simulink model "sim_discrete_7dof"  (R2022b)
settings: Solver=VariableStepAuto  StartTime=0.0  StopTime=T_sim  FixedStep=param_global.Ta  RelTol=1e-3
InitFcn:
  | parameters_7dof;
undefined symbols (not defined in the file): fx, fy, fz, init_bus_param, MPC9, n, param_global, param_robot, param_savgol, param_vis, tau_x, tau_y, tau_z, v4_kin_int_refsys
settings Model: Creator=emu  LastModifiedBy=emu
settings OptimizationCC: ReuseModelBlockBuffer=on
settings DebuggingCC: ReadBeforeWriteMsg=DisableAll  WriteAfterWriteMsg=DisableAll  WriteAfterReadMsg=DisableAll  MultiTaskDSMMsg=none
settings ModelReferenceCC: UpdateModelReferenceTargets=IfOutOfDate
settings SFSimCC: SFSimEcho=off
settings ExplorerConfigSet: InternalSimMechanicsExplorerSettings="<ExplorerConfiguration><canonicalview>default</canonicalview><AnimationSetting><BasePlaybackSpeed>1.0</BasePlaybackSpeed><PlaybackSpeedFactor>1.0</PlaybackSpeedFactor></AnimationSetting><TilePanel><TileInfo><Tiles Columns=\"1\" Count=\"1\" Rows=\"1\"><Column Weight=\"1\"/><Row Weight=\"1\"/><Tile Height=\"1\" Width=\"1\" X=\"0\" Y=\"0\"/></Tiles></TileInfo><SceneInfo><SceneViewer><BGColor><R>0.60000002384185791</R><G>0.60000002384185791</G><B>0.60000002384185791</B></BGColor><Camera><DoPerspective>off</DoPerspective><Position><X>0.252311079271715533</X><Y>1.1744281053543093</Y><Z>0.804106796949367042</Z></Position><Center><X>0.252311079271715533</X><Y>0.174428105354309249</Y><Z>0.804106796949367042</Z></Center><Up><X>0</X><Y>0</Y><Z>1</Z></Up><ViewLimDist>1</ViewLimDist><YLim>0.464787140947337862</YLim><XLim>0.887662117098616976</XLim></Camera></SceneViewer></SceneInfo></TilePanel><MechEditorPanel><Cameras/><GfxPanelCameraMap/><VideoCreator><PlaybackSpeedRatio>1.0</PlaybackSpeedRatio><FrameRate>30</FrameRate><VideoFormat>Motion JPEG AVI</VideoFormat><FrameSize>auto</FrameSize></VideoCreator></MechEditorPanel></ExplorerConfiguration>"

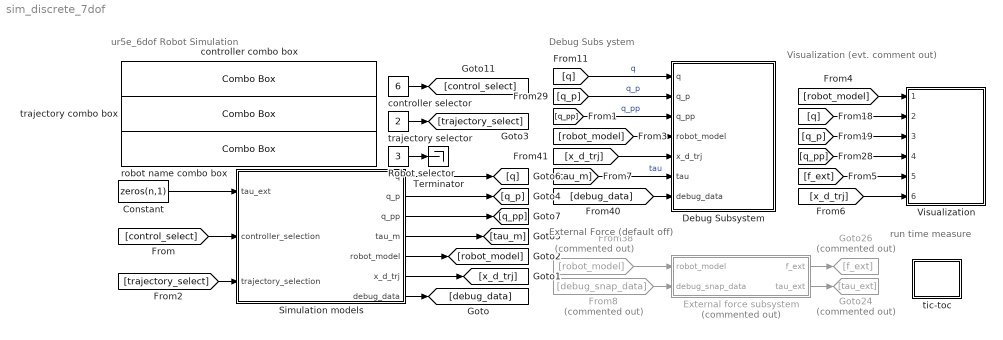
== system sim_discrete_7dof ==
  note: run time measure
  note: ur5e_6dof Robot Simulation
  note: Visualization (evt. comment out)
  note: Debug Subs ystem
  note: External Force (default off)
  Constant : Constant  Value=zeros(n,1)
  Debug Subsystem : Subsystem
  External force subsystem : Subsystem  Commented=on
  From38 : From  Commented=on  GotoTag=robot_model
  From8 : From  Commented=on  GotoTag=debug_snap_data
  Goto24 : Goto  Commented=on  GotoTag=tau_ext
  Goto26 : Goto  Commented=on  GotoTag=f_ext
  Robot selector : Constant  Value=3
  Simulation models : Subsystem
  Terminator : Terminator
  Visualization : Subsystem  ReferencedSubsystem=Visualization_shared_subsystem
  controller combo box : ComboBox  SelectedLabel=MPC9 (v4_kin_int_refsys)
      settings: Values={{'Cartesian CT Control', 'MPC01', 'MPC6 (v3_quat)', 'MPC7 (v3_rpy)', 'MPC8 (v4_kin_int)', 'MPC9 (v4_kin_int_refsys)', 'MPC10 (v5_kin_dev)'}, [1 2 3 4 5 6 7]}
  controller selector : Constant  Value=6  OutDataTypeStr=uint32  SampleTime=-1
  robot name combo box : ComboBox  SelectedLabel=ur5e_6dof
      settings: Values={{'fr3_7dof', 'fr3_6dof', 'ur5e_6dof'}, [1 2 3]}
  tic-toc : Subsystem
  trajectory combo box : ComboBox  SelectedLabel=2: Allsingularity, Polynomial, Workspace
      settings: Values={{'1: Wrist Singularity 1, Polynomial, Workspace', '2: Allsingularity, Polynomial, Workspace', '3: Ellbow Singularity 1, Polynomial, Workspace', '4: ELLBOW Singularity 2, Polynomial, Workspace', '5: ELLBOW Singularity 2, Polynomial, joint space', '6: Shoulder Singularity, Polynomial, Workspace', '7: Shoulder Sing 2, Polynomial, Workspace'}, [1 2 3 4 5 6 7]}
  trajectory selector : Constant  Value=2  OutDataTypeStr=uint32  SampleTime=-1
  wires:
  controller selector/1 -> [control_select]
  [tau_m] -> Debug Subsystem/6(tau)  "tau"
  [debug_data] -> Debug Subsystem/7(debug_data)
  External force subsystem/1(f_ext) -> Goto26/1
  [q_p] -> Debug Subsystem/2(q_p)  "q_p"
  [robot_model] -> Debug Subsystem/4(robot_model)
  [robot_model] -> Visualization/1
  From8/1 -> External force subsystem/2(debug_snap_data)
  [q_pp] -> Visualization/4
  [f_ext] -> Visualization/5
  [x_d_trj] -> Debug Subsystem/5(x_d_trj)
  From38/1 -> External force subsystem/1(robot_model)
  [q_p] -> Visualization/3
  External force subsystem/2(tau_ext) -> Goto24/1
  [q] -> Visualization/2
  [q] -> Debug Subsystem/1(q)  "q"
  [q_pp] -> Debug Subsystem/3(q_pp)  "q_pp"
  Simulation models/7(debug_data) -> [debug_data]
  Simulation models/6(x_d_trj) -> [x_d_trj]
  Simulation models/5(robot_model) -> [robot_model]
  Simulation models/4(tau_m) -> [tau_m]
  Simulation models/3(q_pp) -> [q_pp]
  Simulation models/2(q_p) -> [q_p]
  Simulation models/1(q) -> [q]
  [control_select] -> Simulation models/2(controller_selection)
  Constant/1 -> Simulation models/1(tau_ext)
  trajectory selector/1 -> [trajectory_select]
  [trajectory_select] -> Simulation models/3(trajectory_selection)
  Robot selector/1 -> Terminator/1
  [x_d_trj] -> Visualization/6

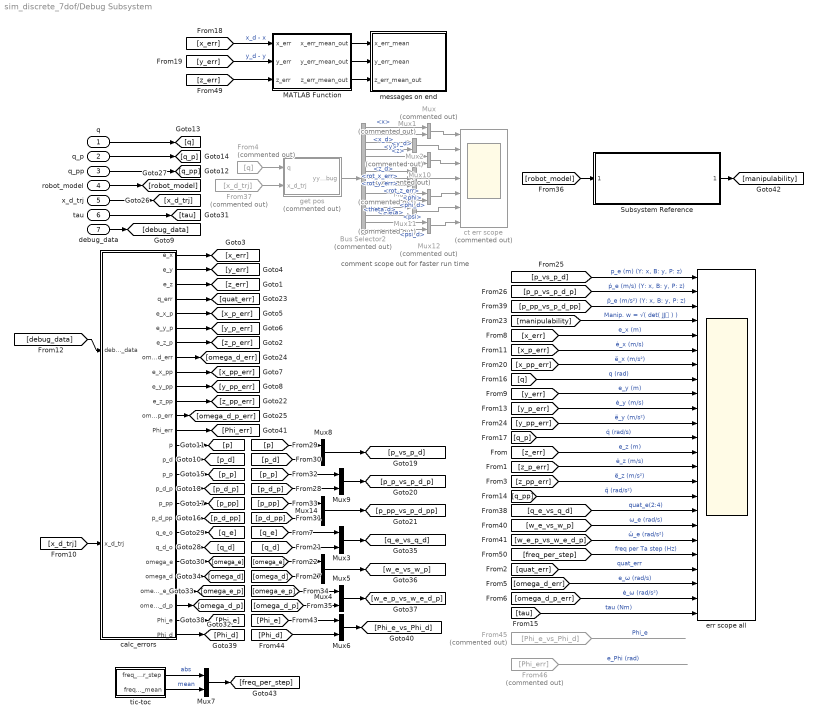
== system sim_discrete_7dof/Debug Subsystem ==
  note: comment scope out for faster run time
  q : Inport
  q_p : Inport  Port=2
  q_pp : Inport  Port=3
  robot_model : Inport  Port=4
  x_d_trj : Inport  Port=5
  tau : Inport  Port=6
  debug_data : Inport  Port=7  OutDataTypeStr=Bus: debug_data_bus
  Bus Selector2 : BusSelector  Commented=on  OutputSignals=x,x_d,y,y_d,z,z_d,rot_x_err,rot_y_err,rot_z_err,phi,phi_d,theta,theta_d,psi,psi_d
  From37 : From  Commented=on  GotoTag=x_d_trj
  From4 : From  Commented=on  GotoTag=q
  From45 : From  Commented=on  GotoTag=Phi_e_vs_Phi_d
  From46 : From  Commented=on  GotoTag=Phi_err
  MATLAB Function : MATLAB Function  TreatAsAtomicUnit=on
  Mux{,1..2,10..12} (6 alike) : Mux  Commented=on  Inputs=2
  Mux13 : Mux  Commented=on  Inputs=3
  Mux{3..9,14} (8 alike) : Mux  Inputs=2
  Subsystem Reference : Subsystem  ReferencedSubsystem=manipulability_and_collinearity
  calc_errors : MATLAB Function  TreatAsAtomicUnit=on
  ct err scope : Scope  Commented=on  NumInputPorts=7
  err scope all : Scope  NumInputPorts=24
  get pos : MATLAB Function  Commented=on  TreatAsAtomicUnit=on  SystemSampleTime=param_global.Ta
  messages on end : Subsystem
  tic-toc : Subsystem
  wires:
  q/1 -> [q]
  q_p/1 -> [q_p]
  q_pp/1 -> [q_pp]
  From4/1 -> get pos/1(q)
  x_d_trj/1 -> [x_d_trj]
  robot_model/1 -> [robot_model]
  debug_data/1 -> [debug_data]
  tau/1 -> [tau]
  From37/1 -> get pos/2(x_d_trj)
  get pos/1(yy_debug) -> Bus Selector2/1
  Mux/1 -> ct err scope/1
  Mux1/1 -> ct err scope/2
  Mux2/1 -> ct err scope/3
  Mux10/1 -> ct err scope/5
  Mux11/1 -> ct err scope/6
  Mux12/1 -> ct err scope/7
  Mux13/1 -> ct err scope/4
  Bus Selector2/1 -> Mux/1  "<x>"
  Bus Selector2/2 -> Mux/2  "<x_d>"
  Bus Selector2/3 -> Mux1/1  "<y>"
  Bus Selector2/4 -> Mux1/2  "<y_d>"
  Bus Selector2/5 -> Mux2/1  "<z>"
  Bus Selector2/6 -> Mux2/2  "<z_d>"
  Bus Selector2/7 -> Mux13/1  "<rot_x_err>"
  Bus Selector2/8 -> Mux13/2  "<rot_y_err>"
  Bus Selector2/9 -> Mux13/3  "<rot_z_err>"
  Bus Selector2/10 -> Mux10/1  "<phi>"
  Bus Selector2/11 -> Mux10/2  "<phi_d>"
  Bus Selector2/12 -> Mux11/1  "<theta>"
  Bus Selector2/13 -> Mux11/2  "<theta_d>"
  Bus Selector2/14 -> Mux12/1  "<psi>"
  Bus Selector2/15 -> Mux12/2  "<psi_d>"
  [x_err] -> MATLAB Function/1(x_err)  "x_d - x"
  [y_err] -> MATLAB Function/2(y_err)  "y_d - y"
  MATLAB Function/2(y_err_mean_out) -> messages on end/2(y_err_mean)
  MATLAB Function/1(x_err_mean_out) -> messages on end/1(x_err_mean)
  [debug_data] -> calc_errors/1(debug_data)
  [x_d_trj] -> calc_errors/2(x_d_trj)
  calc_errors/1(e_x) -> [x_err]
  calc_errors/2(e_y) -> [y_err]
  calc_errors/5(e_x_p) -> [x_p_err]
  calc_errors/6(e_y_p) -> [y_p_err]
  calc_errors/9(e_x_pp) -> [x_pp_err]
  calc_errors/10(e_y_pp) -> [y_pp_err]
  [manipulability] -> err scope all/4  "Manip. w = √( det( JJ⸆ ) )"
  [tau] -> err scope all/24  "tau (Nm)"
  [x_err] -> err scope all/5  "e_x (m)"
  [y_err] -> err scope all/9  "e_y (m)"
  [x_p_err] -> err scope all/6  "ė_x (m/s)"
  [y_p_err] -> err scope all/10  "ė_y (m/s)"
  [x_pp_err] -> err scope all/7  "ё_x (m/s²)"
  [y_pp_err] -> err scope all/11  "ё_y (m/s²)"
  [q] -> err scope all/8  "q (rad)"
  [q_p] -> err scope all/12  "q̇ (rad/s)"
  [q_pp] -> err scope all/16  "q̈ (rad/s²)"
  [p_d_p] -> Mux9/2
  [p_p] -> Mux9/1
  [p_d] -> Mux8/2
  [p] -> Mux8/1
  [p_pp] -> Mux14/1
  [p_d_pp] -> Mux14/2
  [p_p_vs_p_d_p] -> err scope all/2  "ṗ_e (m/s) (Y: x, B: y, P: z)"
  [p_vs_p_d] -> err scope all/1  "p_e (m) (Y: x, B: y, P: z)"
  [p_pp_vs_p_d_pp] -> err scope all/3  "p̈_e (m/s²) (Y: x, B: y, P: z)"
  Mux8/1 -> [p_vs_p_d]
  Mux9/1 -> [p_p_vs_p_d_p]
  Mux14/1 -> [p_pp_vs_p_d_pp]
  calc_errors/14(p) -> [p]
  calc_errors/15(p_d) -> [p_d]
  calc_errors/16(p_p) -> [p_p]
  calc_errors/17(p_d_p) -> [p_d_p]
  calc_errors/18(p_pp) -> [p_pp]
  calc_errors/19(p_d_pp) -> [p_d_pp]
  calc_errors/3(e_z) -> [z_err]
  calc_errors/7(e_z_p) -> [z_p_err]
  calc_errors/11(e_z_pp) -> [z_pp_err]
  [z_err] -> err scope all/13  "e_z (m)"
  [z_p_err] -> err scope all/14  "ė_z (m/s)"
  [z_pp_err] -> err scope all/15  "ё_z (m/s²)"
  calc_errors/4(q_err) -> [quat_err]
  calc_errors/12(omega_d_p_err) -> [omega_d_p_err]
  calc_errors/8(omega_d_err) -> [omega_d_err]
  [quat_err] -> err scope all/21  "quat_err"
  [omega_d_err] -> err scope all/22  "e_ω (rad/s)"
  [omega_d_p_err] -> err scope all/23  "ė_ω (rad/s²)"
  calc_errors/20(q_e_o) -> [q_e]
  calc_errors/21(q_d_o) -> [q_d]
  calc_errors/22(omega_e) -> [omega_e]
  calc_errors/23(omega_d) -> [omega_d]
  calc_errors/24(omega_e_p) -> [omega_e_p]
  calc_errors/25(omega_d_p) -> [omega_d_p]
  [q_e] -> Mux3/1
  [q_d] -> Mux3/2
  [omega_e] -> Mux4/1
  [omega_d] -> Mux4/2
  [omega_e_p] -> Mux5/1
  [omega_d_p] -> Mux5/2
  Mux3/1 -> [q_e_vs_q_d]
  Mux4/1 -> [w_e_vs_w_p]
  Mux5/1 -> [w_e_p_vs_w_e_d_p]
  [q_e_vs_q_d] -> err scope all/17  "quat_e(2:4)"
  [w_e_vs_w_p] -> err scope all/18  "ω_e (rad/s)"
  [w_e_p_vs_w_e_d_p] -> err scope all/19  "ὠ_e (rad/s²)"
  calc_errors/26(Phi_e) -> [Phi_e]
  calc_errors/27(Phi_d) -> [Phi_d]
  [Phi_d] -> Mux6/2
  [Phi_e] -> Mux6/1
  Mux6/1 -> [Phi_e_vs_Phi_d]
  From45/1 -> ?  "Phi_e"
  calc_errors/13(Phi_err) -> [Phi_err]
  From46/1 -> ?  "e_Phi (rad)"
  [z_err] -> MATLAB Function/3(z_err)
  MATLAB Function/3(z_err_mean_out) -> messages on end/3(z_err_mean_out)
  [freq_per_step] -> err scope all/20  "freq per Ta step (Hz)"
  Subsystem Reference/1 -> [manipulability]
  [robot_model] -> Subsystem Reference/1
  Mux7/1 -> [freq_per_step]
  tic-toc/1(freq_per_step) -> Mux7/1  "abs"
  tic-toc/2(freq_per_step_mean) -> Mux7/2  "mean"

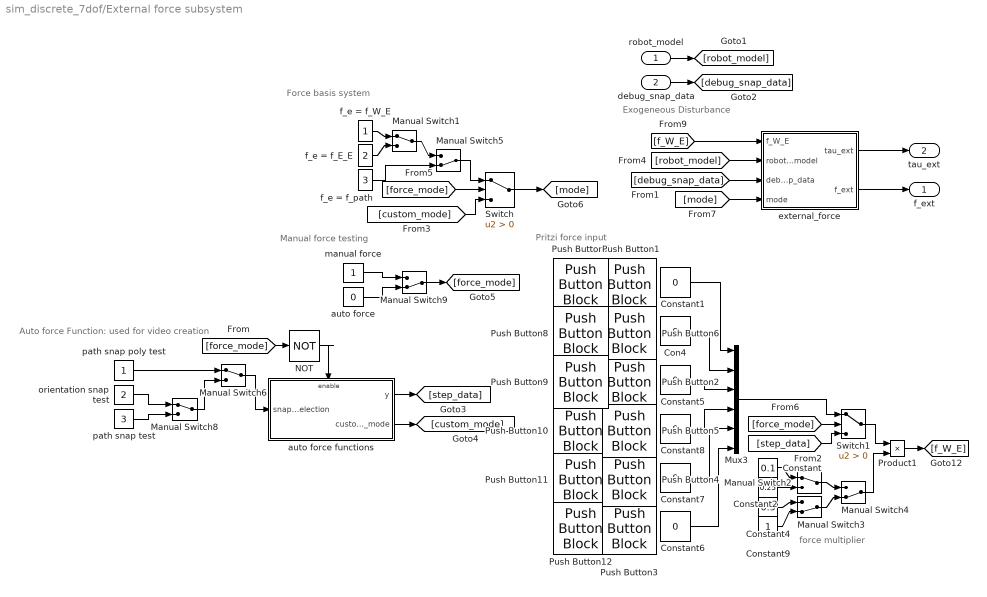
== system sim_discrete_7dof/External force subsystem ==
  note: Force basis system
  note: Manual force testing
  note: Auto force Function: used for video creation
  note: force multiplier
  note: Exogeneous Disturbance
  note: Pritzi force input
  robot_model : Inport
  debug_snap_data : Inport  Port=2  OutDataTypeStr=Bus: debug_snap_data_bus
  Con4 : Constant  Value=0  SampleTime=-1
  Constant : Constant  Value=0.1  SampleTime=-1
  Constant{1,5..8} (5 alike) : Constant  Value=0  SampleTime=-1
  Constant2 : Constant  Value=0.25  SampleTime=-1
  Constant4 : Constant  Value=0.5  SampleTime=-1
  Constant9 : Constant  SampleTime=-1
  Manual Switch{1..2,6,8} (4 alike) : ManualSwitch
  Manual Switch{3..5,9} (4 alike) : ManualSwitch  CurrentSetting=0
  Mux3 : Mux  Inputs=6
  NOT : Logic  Operator=NOT  IconShape=distinctive  AllPortsSameDT=off  OutDataTypeStr=boolean
  Product1 : Product
  Push Button1 : PushButtonBlock  ButtonText=fx  OnValue=20  OffValue=0.000000
  Push Button10 : PushButtonBlock  ButtonText=-tau_x  OnValue=-1  OffValue=0.000000
  Push Button11 : PushButtonBlock  ButtonText=-tau_y  OnValue=-1  OffValue=0.000000
  Push Button12 : PushButtonBlock  ButtonText=-tau_z  OnValue=-1  OffValue=0.000000
  Push Button2 : PushButtonBlock  ButtonText=fz  OnValue=20  OffValue=0.000000
  Push Button3 : PushButtonBlock  ButtonText=tau_z  OffValue=0.000000
  Push Button4 : PushButtonBlock  ButtonText=tau_y  OffValue=0.000000
  Push Button5 : PushButtonBlock  ButtonText=tau_x  OffValue=0.000000
  Push Button6 : PushButtonBlock  ButtonText=fy  OnValue=20  OffValue=0.000000
  Push Button7 : PushButtonBlock  ButtonText=-fx  OnValue=-20  OffValue=0.000000
  Push Button8 : PushButtonBlock  ButtonText=-fy  OnValue=-20  OffValue=0.000000
  Push Button9 : PushButtonBlock  ButtonText=-fz  OnValue=-20  OffValue=0.000000
  Switch : Switch  Criteria=u2 > Threshold  SaturateOnIntegerOverflow=off  InputSameDT=off
  Switch1 : Switch  Criteria=u2 > Threshold  SaturateOnIntegerOverflow=off  InputSameDT=off
  auto force : Constant  Value=0
  auto force functions : Subsystem
  external_force : MATLAB Function  TreatAsAtomicUnit=on
  f_e = f_E_E : Constant  Value=2  SampleTime=-1
  f_e = f_W_E : Constant  SampleTime=-1
  f_e = f_path : Constant  Value=3  SampleTime=-1
  manual force : Constant
  orientation snap test : Constant  Value=2
  path snap poly test : Constant
  path snap test : Constant  Value=3
  f_ext : Outport
  tau_ext : Outport  Port=2
  wires:
  Product1/1 -> [f_W_E]
  Constant4/1 -> Manual Switch3/1
  Constant6/1 -> Mux3/6
  Constant5/1 -> Mux3/3
  Constant/1 -> Manual Switch2/1
  Constant8/1 -> Mux3/4
  [f_W_E] -> external_force/1(f_W_E)
  external_force/2(f_ext) -> f_ext/1
  Constant9/1 -> Manual Switch3/2
  Manual Switch2/1 -> Manual Switch4/1
  Con4/1 -> Mux3/2
  [robot_model] -> external_force/2(robot_model)
  Manual Switch4/1 -> Product1/2
  Constant1/1 -> Mux3/1
  f_e = f_W_E/1 -> Manual Switch1/1
  Constant7/1 -> Mux3/5
  Constant2/1 -> Manual Switch2/2
  f_e = f_E_E/1 -> Manual Switch1/2
  Manual Switch3/1 -> Manual Switch4/2
  external_force/1(tau_ext) -> tau_ext/1
  Manual Switch1/1 -> Manual Switch5/1
  f_e = f_path/1 -> Manual Switch5/2
  robot_model/1 -> [robot_model]
  debug_snap_data/1 -> [debug_snap_data]
  [debug_snap_data] -> external_force/3(debug_snap_data)
  Switch1/1 -> Product1/1
  Manual Switch5/1 -> Switch/1
  [custom_mode] -> Switch/3
  auto force functions/1(y) -> [step_data]
  auto force functions/2(custom_mode) -> [custom_mode]
  Manual Switch6/1 -> auto force functions/1(snap selection)
  path snap test/1 -> Manual Switch8/2
  orientation snap test/1 -> Manual Switch8/1
  manual force/1 -> Manual Switch9/1
  auto force/1 -> Manual Switch9/2
  Manual Switch9/1 -> [force_mode]
  [force_mode] -> Switch/2
  [force_mode] -> Switch1/2
  [step_data] -> Switch1/3
  Mux3/1 -> Switch1/1
  Switch/1 -> [mode]
  [mode] -> external_force/4(mode)
  Manual Switch8/1 -> Manual Switch6/2
  path snap poly test/1 -> Manual Switch6/1
  [force_mode] -> NOT/1
  NOT/1 -> auto force functions/Enable

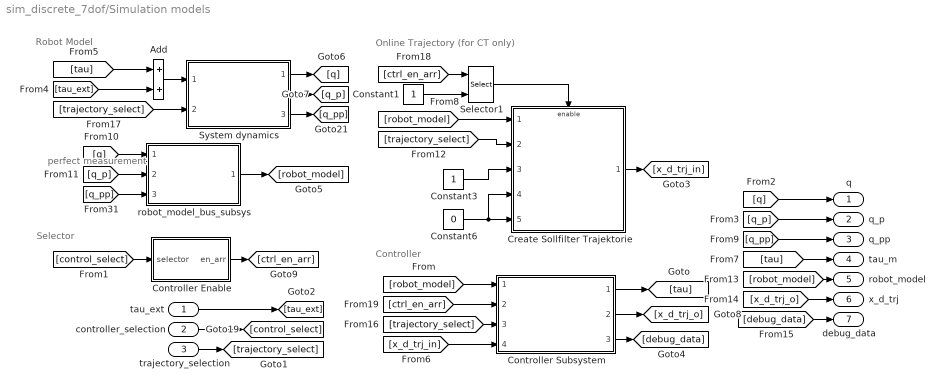
== system sim_discrete_7dof/Simulation models ==
  note: Selector
  note: Controller
  note: Online Trajectory (for CT only)
  note: Robot Model
  note: perfect measurement
  tau_ext : Inport
  controller_selection : Inport  Port=2
  trajectory_selection : Inport  Port=3
  Add : Sum
  Constant1 : Constant
  Constant3 : Constant
  Constant6 : Constant  Value=0
  Controller Enable : MATLAB Function  TreatAsAtomicUnit=on
  Controller Subsystem : Subsystem  ReferencedSubsystem=controller_ref_subsys
  Create Sollfilter Trajektorie : Subsystem  ReferencedSubsystem=trajectory_generation_ref_subsys_7dof
  Selector1 : Selector  IndexOptions=Index vector (port)  Indices=[1 3]  OutputSizes=1
  System dynamics : Subsystem  ReferencedSubsystem=robot_model_7dof_ref_subsys
  robot_model_bus_subsys : Subsystem  ReferencedSubsystem=robot_model_bus_7dof_ref_subsys
  q : Outport
  q_p : Outport  Port=2
  q_pp : Outport  Port=3
  tau_m : Outport  Port=4
  robot_model : Outport  Port=5  OutDataTypeStr=Bus: robot_model
  x_d_trj : Outport  Port=6  OutDataTypeStr=Bus: x_d
  debug_data : Outport  Port=7  OutDataTypeStr=Bus: debug_data_bus
  wires:
  [q_p] -> robot_model_bus_subsys/2
  System dynamics/2 -> [q_p]
  [tau_ext] -> Add/2
  System dynamics/3 -> [q_pp]
  [q] -> robot_model_bus_subsys/1
  [q_pp] -> robot_model_bus_subsys/3
  System dynamics/1 -> [q]
  [robot_model] -> Create Sollfilter Trajektorie/1
  robot_model_bus_subsys/1 -> [robot_model]
  tau_ext/1 -> [tau_ext]
  controller_selection/1 -> [control_select]
  [q_pp] -> q_pp/1
  [q_p] -> q_p/1
  [x_d_trj_o] -> x_d_trj/1
  [debug_data] -> debug_data/1
  [q] -> q/1
  [robot_model] -> robot_model/1
  Constant3/1 -> Create Sollfilter Trajektorie/3
  Constant6/1 -> Create Sollfilter Trajektorie/4, Create Sollfilter Trajektorie/5
  Create Sollfilter Trajektorie/1 -> [x_d_trj_in]
  trajectory_selection/1 -> [trajectory_select]
  [trajectory_select] -> Create Sollfilter Trajektorie/2
  Add/1 -> System dynamics/1
  [tau] -> tau_m/1
  [tau] -> Add/1
  Controller Subsystem/3 -> [debug_data]
  Controller Subsystem/2 -> [x_d_trj_o]
  Controller Subsystem/1 -> [tau]
  [robot_model] -> Controller Subsystem/1
  [x_d_trj_in] -> Controller Subsystem/4
  [trajectory_select] -> Controller Subsystem/3
  [control_select] -> Controller Enable/1(selector)
  Controller Enable/1(en_arr) -> [ctrl_en_arr]
  [ctrl_en_arr] -> Selector1/1
  Selector1/1 -> Create Sollfilter Trajektorie/Enable
  Constant1/1 -> Selector1/2
  [ctrl_en_arr] -> Controller Subsystem/2
  [trajectory_select] -> System dynamics/2

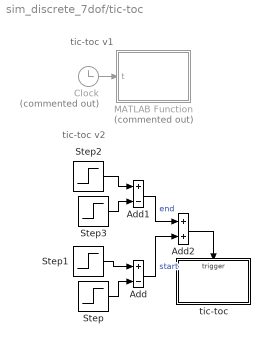
== system sim_discrete_7dof/tic-toc ==
  note: tic-toc v1
  note: tic-toc v2
  Add : Sum  Inputs=+-
  Add1 : Sum  Inputs=+-
  Add2 : Sum
  Clock : Clock  Commented=on
  MATLAB Function : MATLAB Function  Commented=on  TreatAsAtomicUnit=on
  Step : Step  Time=param_global.Ta*2  SampleTime=param_global.Ta
  Step1 : Step  Time=param_global.Ta  SampleTime=param_global.Ta
  Step2 : Step  Time=param_vis.T-param_global.Ta  SampleTime=param_global.Ta
  Step3 : Step  Time=param_vis.T  SampleTime=param_global.Ta
  tic-toc : Subsystem  TreatAsAtomicUnit=on
  wires:
  Add/1 -> Add2/2  "start"
  Step2/1 -> Add1/1
  Add2/1 -> tic-toc/Trigger
  Step3/1 -> Add1/2
  Add1/1 -> Add2/1  "end"
  Step1/1 -> Add/1
  Step/1 -> Add/2
  Clock/1 -> MATLAB Function/1(t)

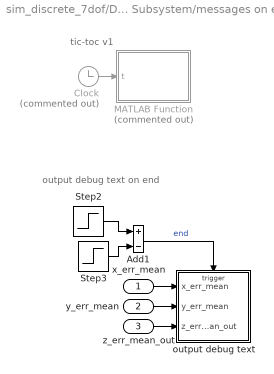
== system sim_discrete_7dof/Debug Subsystem/messages on end ==
  note: tic-toc v1
  note: output debug text on end
  x_err_mean : Inport
  y_err_mean : Inport  Port=2
  z_err_mean_out : Inport  Port=3
  Add1 : Sum  Inputs=+-
  Clock : Clock  Commented=on
  MATLAB Function : MATLAB Function  Commented=on  TreatAsAtomicUnit=on
  Step2 : Step  Time=param_vis.T-param_global.Ta  SampleTime=param_global.Ta
  Step3 : Step  Time=param_vis.T  SampleTime=param_global.Ta
  output debug text : Subsystem  TreatAsAtomicUnit=on
  wires:
  Clock/1 -> MATLAB Function/1(t)
  Add1/1 -> output debug text/Trigger  "end"
  Step3/1 -> Add1/2
  Step2/1 -> Add1/1
  y_err_mean/1 -> output debug text/2(y_err_mean)
  x_err_mean/1 -> output debug text/1(x_err_mean)
  z_err_mean_out/1 -> output debug text/3(z_err_mean_out)

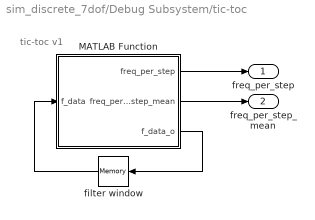
== system sim_discrete_7dof/Debug Subsystem/tic-toc ==
  note: tic-toc v1
  MATLAB Function : MATLAB Function  TreatAsAtomicUnit=on
  filter window : Memory  InitialCondition=zeros(param_savgol.N, 1)
  freq_per_step : Outport
  freq_per_step_mean : Outport  Port=2
  wires:
  MATLAB Function/1(freq_per_step) -> freq_per_step/1
  filter window/1 -> MATLAB Function/1(f_data)
  MATLAB Function/2(freq_per_step_mean) -> freq_per_step_mean/1
  MATLAB Function/3(f_data_o) -> filter window/1

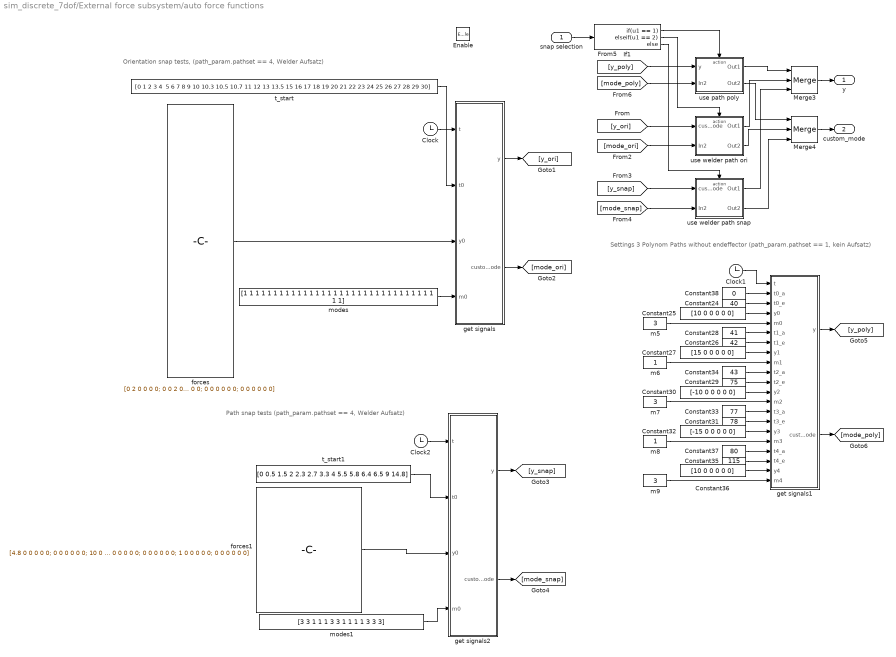
== system sim_discrete_7dof/External force subsystem/auto force functions ==
  note: Orientation snap tests, (path_param.pathset == 4, Welder Aufsatz)
  note: Path snap tests (path_param.pathset == 4, Welder Aufsatz)
  note: Settings 3 Polynom Paths without endeffector
      | (path_param.pathset == 1, kein Aufsatz)
  snap selection : Inport
  Enable : EnablePort
  Clock : Clock
  Clock1 : Clock
  Clock2 : Clock
  Constant24 : Constant  Value=40
  Constant25 : Constant  Value=[10 0 0 0 0 0]
  Constant26 : Constant  Value=42
  Constant27 : Constant  Value=[15 0 0 0 0 0]
  Constant28 : Constant  Value=41
  Constant29 : Constant  Value=75
  Constant30 : Constant  Value=[-10 0 0 0 0 0]
  Constant31 : Constant  Value=78
  Constant32 : Constant  Value=[-15 0 0 0 0 0]
  Constant33 : Constant  Value=77
  Constant34 : Constant  Value=43
  Constant35 : Constant  Value=115
  Constant36 : Constant  Value=[10 0 0 0 0 0]
  Constant37 : Constant  Value=80
  Constant38 : Constant  Value=0
  If1 : If  IfExpression=u1 == 1  ElseIfExpressions=u1 == 2
  Merge3 : Merge  Inputs=3
  Merge4 : Merge  Inputs=3
  forces : Constant  Value=|
      | [0 2 0 0 0 0;
      | 0 0 2 0 0 0;
      | 0 -2 0 0 0 0;
      | 0 0 -2 0 0 0;
      | 30 0 7 0 0 0;
      | 0 2 0 0 0 0;
      | 0 0 2 0 0 0;
      | 0 -2 0 0 0 0;
      | 0 0 -2 0 0 0;
      | 0 0 0 0 0 0;
      | 0 0 0 0.25 0 0;
      | 0 0 0 0.26 0 0;
      | 0 0 0 0.27 0 0;
      | 0 0 0 0 0 0;
      | 0 -2 0 0 0 0;
      | 0 0 0 0 0 0;
      | 0 0 0 0.26 0 0;
      | 0 0 0 0 0 0;
      | 0 -2 0 0 0 0;
      | 0 0 2 0 0 0;
      | 0 2 0 0 0 0;
      | 0 0 -2 0 0 0;
      | -30 3.5 -3.5 0 0 0;
      | 0 -2 0 0 0 0;
      | 0 0 2 0 0 0;
      | 0 2 0 0 0 0;
      | 0 0 -2 0 0 0;
      | 0 0 0 0 0 0;
      | 0 0 0 0 0 0;
      | 0 0 0 0 0 0;
      | 0 0 0 0 0 0;
      | 0 0 0 0 0 0;
      | 0 0 0 0 0 0;
      | 0 0 0 0 0 0]
  forces1 : Constant  Value=|
      | [4.8 0 0 0 0 0;
      | 0 0 0 0 0 0;
      | 10 0 0 0 0 0;
      | 15 0 3 0 0 0
      | 10 0 3 0 0 0;
      | 0 0 0 0 0 0;
      | 1 0 0 0 0 0;
      | 0 0 0 0 0 0;
      | 15 0 0 0 0 0;
      | 10 -3 0 0 0 0
      | 10 0 0 0 0 0;
      | 0 0 0 0 0 0;
      | 1 0 0 0 0 0;
      | 0 0 0 0 0 0]
  get signals : MATLAB Function  TreatAsAtomicUnit=on
  get signals1 : MATLAB Function  TreatAsAtomicUnit=on
  get signals2 : MATLAB Function  TreatAsAtomicUnit=on
  m5 : Constant  Value=3
  m6 : Constant
  m7 : Constant  Value=3
  m8 : Constant
  m9 : Constant  Value=3
  modes : Constant  Value=[1 1 1 1 1 1 1 1 1 1 1 1 1 1 1 1 1 1 1 1 1 1 1 1 1 1 1 1 1 1 1 1 1 1]
  modes1 : Constant  Value=[3 3 1 1 1 3 3 1 1 1 1 3 3 3]
  t_start : Constant  Value="[0 1 2 3 4  5 6 7 8 9 10 10.3 10.5 10.7 11 12 13 13.5 15 16 17 18 19 20 21 22 23 24 25 26 27 28 29 30]"
  t_start1 : Constant  Value="[0 0.5 1.5 2 2.3  2.7 3.3 4 5.5  5.8 6.4 6.5 9 14.8]"
  use path poly : Subsystem  TreatAsAtomicUnit=on
  use welder path ori : Subsystem  TreatAsAtomicUnit=on
  use welder path snap : Subsystem  TreatAsAtomicUnit=on
  y : Outport
  custom_mode : Outport  Port=2
  wires:
  Constant26/1 -> get signals1/7(t1_e)
  Constant36/1 -> get signals1/20(y4)
  Constant34/1 -> get signals1/10(t2_a)
  Constant29/1 -> get signals1/11(t2_e)
  Constant37/1 -> get signals1/18(t4_a)
  Constant33/1 -> get signals1/14(t3_a)
  Constant35/1 -> get signals1/19(t4_e)
  Clock/1 -> get signals/1(t)
  m5/1 -> get signals1/5(m0)
  m8/1 -> get signals1/17(m3)
  m7/1 -> get signals1/13(m2)
  m9/1 -> get signals1/21(m4)
  Constant32/1 -> get signals1/16(y3)
  Clock1/1 -> get signals1/1(t)
  m6/1 -> get signals1/9(m1)
  Constant25/1 -> get signals1/4(y0)
  Constant38/1 -> get signals1/2(t0_a)
  Constant31/1 -> get signals1/15(t3_e)
  Constant28/1 -> get signals1/6(t1_a)
  Constant27/1 -> get signals1/8(y1)
  Constant24/1 -> get signals1/3(t0_e)
  Constant30/1 -> get signals1/12(y2)
  use path poly/1(Out1) -> Merge3/1
  use welder path ori/1(Out1) -> Merge3/2
  use path poly/2(Out2) -> Merge4/1
  use welder path ori/2(Out2) -> Merge4/2
  Merge4/1 -> custom_mode/1
  Merge3/1 -> y/1
  If1/1 -> use path poly/Action
  t_start/1 -> get signals/2(t0)
  forces/1 -> get signals/3(y0)
  modes/1 -> get signals/4(m0)
  t_start1/1 -> get signals2/2(t0)
  forces1/1 -> get signals2/3(y0)
  modes1/1 -> get signals2/4(m0)
  Clock2/1 -> get signals2/1(t)
  snap selection/1 -> If1/1
  If1/2 -> use welder path ori/Action
  If1/3 -> use welder path snap/Action
  use welder path snap/1(Out1) -> Merge3/3
  use welder path snap/2(Out2) -> Merge4/3
  get signals1/1(y) -> [y_poly]
  get signals1/2(custom_mode) -> [mode_poly]
  get signals2/1(y) -> [y_snap]
  get signals2/2(custom_mode) -> [mode_snap]
  get signals/1(y) -> [y_ori]
  get signals/2(custom_mode) -> [mode_ori]
  [y_poly] -> use path poly/1(y)
  [mode_poly] -> use path poly/2(In2)
  [y_ori] -> use welder path ori/1(custom_mode)
  [mode_ori] -> use welder path ori/2(In2)
  [y_snap] -> use welder path snap/1(custom_mode)
  [mode_snap] -> use welder path snap/2(In2)

== system sim_discrete_7dof/tic-toc/tic-toc ==
  Trigger : TriggerPort  VariantControl=(inherit)
  MATLAB Function : MATLAB Function  TreatAsAtomicUnit=on

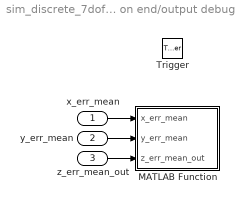
== system sim_discrete_7dof/Debug Subsystem/messages on end/output debug text ==
  x_err_mean : Inport
  y_err_mean : Inport  Port=2
  z_err_mean_out : Inport  Port=3
  Trigger : TriggerPort  VariantControl=(inherit)
  MATLAB Function : MATLAB Function  TreatAsAtomicUnit=on
  wires:
  y_err_mean/1 -> MATLAB Function/2(y_err_mean)
  x_err_mean/1 -> MATLAB Function/1(x_err_mean)
  z_err_mean_out/1 -> MATLAB Function/3(z_err_mean_out)

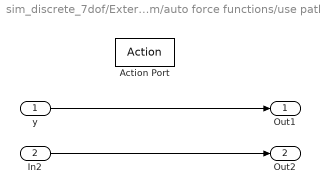
== system sim_discrete_7dof/External force subsystem/auto force functions/use path poly ==
  y : Inport
  In2 : Inport  Port=2
  Action Port : ActionPort
  Out1 : Outport
  Out2 : Outport  Port=2
  wires:
  In2/1 -> Out2/1
  y/1 -> Out1/1

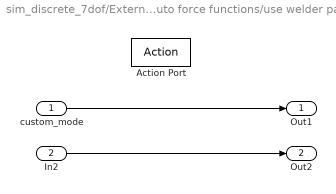
== system sim_discrete_7dof/External force subsystem/auto force functions/use welder path ori ==
  custom_mode : Inport
  In2 : Inport  Port=2
  Action Port : ActionPort
  Out1 : Outport
  Out2 : Outport  Port=2
  wires:
  custom_mode/1 -> Out1/1
  In2/1 -> Out2/1

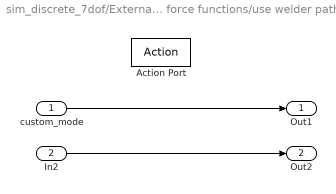
== system sim_discrete_7dof/External force subsystem/auto force functions/use welder path snap ==
  custom_mode : Inport
  In2 : Inport  Port=2
  Action Port : ActionPort
  Out1 : Outport
  Out2 : Outport  Port=2
  wires:
  In2/1 -> Out2/1
  custom_mode/1 -> Out1/1

== matlab function sim_discrete_7dof/Simulation models/Controller Enable ==
  settings: sampleTime=param_global.Ta
  data: en_arr output; selector input uint32
function en_arr  = fcn(selector)
    % Wichtig: selector \in [1,max(selector)]
    % Es wird ein bool array ausgegeben, welches nur den index 1 setzt, der
    % mit selector übereinstimmt. Achtung: Size von "en_arr" muss
    % entsprechend der Ausgänge unter "Edit Data" manuell angegeben werden.
    % Beispiel: 4 Inputs, max(selector)=4, Size = [1 4]
    % z. B. selector = 2
    % 1:4 == selector liefert [0 1 0 0]
    en_arr = (1:7 == selector)';
end

== matlab function sim_discrete_7dof/External force subsystem/auto force functions/get signals ==
  data: t input; y output size=6; t0 input; y0 input; m0 input; custom_mode output
function [y,custom_mode] = fcn(t, t0, y0, m0)
% ti_a ... Anfangszeit
% ti_e ... Endzeit
% yi ... Pulswert
% mi ... mode: 1 if f_w_e, 2 if f_e_e, 3 if f_path
% outputs
% y ... chosen Pulswert
% custom mode: chose mode

i = sum(t >= t0);
y = y0(i,:)';
custom_mode = m0(i);

== matlab function sim_discrete_7dof/External force subsystem/auto force functions/get signals1 ==
  data: t input; y output size=6; t0_a input; t0_e input; y0 input; m0 input; t1_a input; t1_e input; y1 input; m1 input; t2_a input; t2_e input; y2 input; m2 input; t3_a input; t3_e input; y3 input; m3 input; t4_a input; t4_e input; y4 input; custom_mode output; m4 input
function [y,custom_mode] = fcn(t, t0_a, t0_e, y0, m0, t1_a, t1_e, y1, m1, t2_a, t2_e, y2, m2, t3_a, t3_e, y3, m3, t4_a, t4_e, y4, m4)
% ti_a ... Anfangszeit
% ti_e ... Endzeit
% yi ... Pulswert
% mi ... mode: 1 if f_w_e, 2 if f_e_e, 3 if f_path
% outputs
% y ... chosen Pulswert
% custom mode: chose mode

if(t >= t0_a && t < t0_e)
    y = y0;
    custom_mode = m0; % f_path
elseif(t >= t1_a && t < t1_e)
    y = y1;
    custom_mode = m1; % f_e_e
elseif(t >= t2_a && t < t2_e)
    y = y2;
    custom_mode = m2; % f_path
elseif(t >= t3_a && t < t3_e)
    y = y3;
    custom_mode = m3; % f_path
elseif(t >= t4_a && t < t4_e)
    y = y4;
    custom_mode = m4; % f_path
else
    y = [0 0 0 0 0 0]';
    custom_mode = 1; % f_w_e
end

== matlab function sim_discrete_7dof/External force subsystem/auto force functions/get signals2 ==
  data: t input; y output size=6; t0 input; y0 input; m0 input; custom_mode output
function [y,custom_mode] = fcn(t, t0, y0, m0)
% ti_a ... Anfangszeit
% ti_e ... Endzeit
% yi ... Pulswert
% mi ... mode: 1 if f_w_e, 2 if f_e_e, 3 if f_path
% outputs
% y ... chosen Pulswert
% custom mode: chose mode

i = sum(t >= t0);
y = y0(i,:)';
custom_mode = m0(i);

== matlab function sim_discrete_7dof/tic-toc/MATLAB Function ==
  settings: updateMethod=DISCRETE  sampleTime=param_global.Ta
  data: t input; param_vis parameter
function fcn(t, param_vis)

if(t==0)
    tic;
end

if(t==param_vis.T)
    toc;
end

== matlab function sim_discrete_7dof/Debug Subsystem/messages on end/MATLAB Function ==
  settings: updateMethod=DISCRETE  sampleTime=param_global.Ta
  data: t input; param_vis parameter
function fcn(t, param_vis)

if(t==0)
    tic;
end

if(t==param_vis.T)
    toc;
end

== matlab function sim_discrete_7dof/tic-toc/tic-toc/MATLAB Function ==
  settings: updateMethod=DISCRETE
function fcn()
persistent flag;

if(isempty(flag))
    flag=0;
end

if(flag == 0)
    tic
    flag=1;
else
    disp(['Simulink execution time: ', sprintf('%f', toc), ' s']);
end

== matlab function sim_discrete_7dof/Debug Subsystem/messages on end/output debug text/MATLAB Function ==
  settings: updateMethod=DISCRETE
  data: x_err_mean input; y_err_mean input; z_err_mean_out input
function fcn(x_err_mean, y_err_mean, z_err_mean_out)
    disp(['mean x_err = ', sprintf('%g', x_err_mean),     ' m']);
    disp(['mean y_err = ', sprintf('%g', y_err_mean),     ' m']);
    disp(['mean y_err = ', sprintf('%g', z_err_mean_out), ' m']);
end

== matlab function sim_discrete_7dof/Debug Subsystem/MATLAB Function ==
  data: x_err_mean_out output; x_err input; y_err input; y_err_mean_out output; z_err input; z_err_mean_out output
function [x_err_mean_out, y_err_mean_out, z_err_mean_out] = fcn(x_err, y_err, z_err)

persistent cnt;
persistent x_err_mean;
persistent y_err_mean;
persistent z_err_mean;

if(isempty(cnt))
    cnt = 1;
    x_err_mean = 0;
    y_err_mean = 0;
    z_err_mean = 0;
end
% m1 =  a          = (0*m0+a)/1
% m2 = (a+b)/2     = (1*m1+b)/2
% m3 = (a+b+c)/3   = (2*m2+c)/3
% m4 = (a+b+c+d)/4 = (3*m3+d)/4
% ...
% mi = ((i-1)*m_{i-1})/i; 
x_err_mean = ((cnt-1)*x_err_mean + x_err)/cnt;
y_err_mean = ((cnt-1)*y_err_mean + y_err)/cnt;
z_err_mean = ((cnt-1)*z_err_mean + z_err)/cnt;

x_err_mean_out = x_err_mean;
y_err_mean_out = y_err_mean;
z_err_mean_out = z_err_mean;

cnt = cnt + 1;

%Die iterative Methode ist anfälliger für Rundungsfehler.
%Die iterative Methode kann bei sehr großen Datenmengen numerisch instabil
% werden

== matlab function sim_discrete_7dof/Debug Subsystem/get pos ==
  settings: updateMethod=DISCRETE  sampleTime=param_global.Ta
  data: q input; yy_debug output Bus: yy_debug_bus; param_robot parameter; x_d_trj input Bus: x_d; init_bus_param parameter
function yy_debug  = fcn(q, param_robot, x_d_trj, init_bus_param)

yy_debug = init_bus_param.init_yy_debug_bus;

H = hom_transform_endeffector(q, param_robot);
y_t_W_E = H(1:3,4);
y_t_W_E_d = x_d_trj.p_d;

R_W_E = H(1:3,1:3);
ori_t_W_E = rotm2eul(R_W_E, 'XYZ');
ori_t_W_E_d = rotm2eul(quaternion2rotation(x_d_trj.q_d), 'XYZ');

yy_debug.x =  y_t_W_E(1);
yy_debug.x_d = y_t_W_E_d(1);

yy_debug.y =  y_t_W_E(2);
yy_debug.y_d = y_t_W_E_d(2);

yy_debug.z =  y_t_W_E(3);
yy_debug.z_d = y_t_W_E_d(3);

yy_debug.phi = ori_t_W_E(1);
yy_debug.phi_d = ori_t_W_E_d(1);

yy_debug.theta = ori_t_W_E(2);
yy_debug.theta_d = ori_t_W_E_d(2);

yy_debug.psi = ori_t_W_E(3);
yy_debug.psi_d = ori_t_W_E_d(3);

quat_err = quat_mult(rotation2quaternion(R_W_E), quat_inv(x_d_trj.q_d));
yy_debug.rot_x_err = quat_err(2);
yy_debug.rot_y_err = quat_err(3);
yy_debug.rot_z_err = quat_err(4);

== matlab function sim_discrete_7dof/Debug Subsystem/calc_errors ==
  data: debug_data input Bus: debug_data_bus; e_x output; e_y output; e_z output; q_err output; e_x_p output; e_y_p output; e_z_p output; omega_d_err output; e_x_pp output; e_y_pp output; e_z_pp output; omega_d_p_err output; Phi_err output; x_d_trj input Bus: x_d; p output; p_d output; p_p output; p_d_p output; p_pp output; p_d_pp output; q_e_o output; q_d_o output; omega_e output; omega_d output; omega_e_p output; omega_d_p output; Phi_e output; Phi_d output
function [e_x, e_y, e_z, q_err, e_x_p, e_y_p, e_z_p, omega_d_err, e_x_pp, e_y_pp, e_z_pp, omega_d_p_err, Phi_err, p, p_d, p_p, p_d_p, p_pp, p_d_pp, q_e_o, q_d_o, omega_e, omega_d, omega_e_p, omega_d_p, Phi_e, Phi_d] = fcn(debug_data, x_d_trj)

p    = debug_data.p;
p_p  = debug_data.p_p;
p_pp = debug_data.p_pp;

q_e = debug_data.q;
omega_e = debug_data.omega;
omega_e_p = debug_data.omega_p;

p_d    = x_d_trj.p_d;
p_d_p  = x_d_trj.p_d_p;
p_d_pp = x_d_trj.p_d_pp;

q_d = x_d_trj.q_d;
omega_d = x_d_trj.omega_d;
omega_d_p = x_d_trj.omega_d_p;

q_e_o = q_e(2:4);
q_d_o = q_d(2:4);

e_x    = p_d(1)    - p(1);
e_x_p  = p_d_p(1)  - p_p(1);
e_x_pp = p_d_pp(1) - p_pp(1);

e_y    = p_d(2)    - p(2);
e_y_p  = p_d_p(2)  - p_p(2);
e_y_pp = p_d_pp(2) - p_pp(2);

e_z    = p_d(3)    - p(3);
e_z_p  = p_d_p(3)  - p_p(3);
e_z_pp = p_d_pp(3) - p_pp(3);

%q_err_full = quat_mult(q_e, quat_inv(q_d));
%q_err = q_err_full(2:4);
q_err = debug_data.q_err(2:4);
omega_d_err = omega_e-omega_d;
omega_d_p_err = omega_e_p-omega_d_p;

R_d = x_d_trj.R_d;
R_e = quaternion2rotation(q_e);

Phi_e = debug_data.Phi;
Phi_d = x_d_trj.Phi_d;
Phi_err = rotm2rpy(R_e*R_d');

== matlab function sim_discrete_7dof/Debug Subsystem/tic-toc/MATLAB Function ==
  settings: updateMethod=DISCRETE  sampleTime=param_global.Ta
  data: freq_per_step output; f_data input; freq_per_step_mean output; param_savgol parameter; f_data_o output
function [freq_per_step, freq_per_step_mean, f_data_o] = fcn(f_data, param_savgol)

persistent cnt;
persistent time_start

if(isempty(time_start))
    tic;
    cnt = 0;
    time_start = 0;
end

if(cnt > 1)
    time_end = toc;
    freq_per_step = 1/(time_end - time_start);
    freq_per_step_mean = param_savgol.bT * f_data;
    time_start = time_end;
else
    freq_per_step = 0;
    freq_per_step_mean = 0;
end

if(cnt < param_savgol.N)
    cnt = cnt + 1;
    f_data(cnt:end) = mean([f_data; freq_per_step]);
end

f_data_o = [freq_per_step; f_data(1:end-1, 1)];
%disp(['Simulink execution time: ', sprintf('%f', time_per_step), ' s']);

== matlab function sim_discrete_7dof/External force subsystem/external_force ==
  settings: updateMethod=DISCRETE  sampleTime=param_global.Ta
  data: f_W_E input; robot_model input; debug_snap_data input Bus: debug_snap_data_bus; tau_ext output; mode input; f_ext output
function [tau_ext, f_ext] = fcn(f_W_E, robot_model, debug_snap_data, mode)
    if(mode == 1) % Kraft ist im Weltsystem definiert
        f_ext = f_W_E; %Externe Kraft / Moment in Welt KOS definiert
    elseif(mode == 2) % Externe Kraft / Moment in Endeffektor KOS definiert
        % Rechnet die Kräfte im Weltsystem die auf den Endeffektor um in Kräfte,
        % die im Endeffektorsystem direkt auf den Endeffektor wirken, damit eine
        % intuitiverer Steuerung möglich ist (Der Benutzer legt ja auch die Kräfte
        % aus Sicht des Endeffektorsystem an und nicht aus Sicht des Weltsystems)
        
        R_W_E = robot_model.H(1:3,1:3);
        
        % indizes nicht ganz logisch
        F_W_E = f_W_E(1:3);
        tau_W_E = f_W_E(4:6);
        
        
        F_E_E = R_W_E*F_W_E;
        tau_E_E = R_W_E*tau_W_E;
        
        f_ext = [F_E_E;tau_E_E];
    else % Externe Kraft im Pfadkoordinatensystem des aktiven Pfads
        F_W_E = f_W_E(1:3);
        tau_W_E = f_W_E(4:6);
        active_path_index_t = debug_snap_data.active_path_index_t;
        if(active_path_index_t == 0) % if CT CONTROL TODO: Problem bei orienation snap wenn path index > N_path ist.
            R_W_path = eye(3);
        else
            R_W_path = debug_snap_data.Rot_transport_frame(:,:,active_path_index_t); % only active path
        end

        F_path_E = R_W_path*F_W_E;
        tau_path_E = R_W_path*tau_W_E;
        
        f_ext = [F_path_E;tau_path_E];
    end
    %theta_star = debug_snap_data.theta_star;
    %N_path = param_global.N_path;

    %R_W_path = debug_snap_data.Rot_transport_frame; % all paths
    %path_frame_position = zeros(3,2,N_path);
    %for i=1:1:N_path
    %    [sigma, ~, ~, ~] = eval_path_t(theta_star(i), i, path_param);
    %    path_frame_position(:,:,i) = [sigma rotm2eul(R_W_path(:,:,i), 'XYZ')];
    %end

    J = robot_model.J;
    tau_ext_temp = J' * f_ext;
    tau_ext = tau_ext_temp(3:9);
end
